simulink model "bldc_new_good"  (R2018a)
settings: Solver=FixedStepDiscrete  StartTime=0.0  StopTime=t_l+0.5  RelTol=1e-3  EnableMultiTasking=on
PreLoadFcn:
  | Ts=2e-6;
values from neighbouring files (symbols this model uses):
  r1 = -0.136    [Platforma_algorytm.m]
  r2 = -0.04    [Platforma_algorytm.m]
  t_l = length(right_foot)*dt    [Platforma_algorytm.m]
  t_r = length(left_foot)*dt    [Platforma_algorytm.m]
  w_x = ((60*v*4.29)/r1)/(2*pi*10)    [Platforma_algorytm.m]
  w_y = ((60*v*4.29)/r2)/(2*pi*10)    [Platforma_algorytm.m]
undefined symbols (not defined in the file or in its folder): DiscIntNeverNeededParam, s
libraries: powerlib_meascontrol x4, powerlib x3, electricdrivelib x2, AC7DriveInternalModels x2, simulink x1
Description:
  | Copyright 2008-2018 The MathWorks, Inc.
settings Model: ExtModeAutoUpdateStatusClock=off  Creator=MathWorks  LastModifiedBy=cinek
settings SolverCC: AutoInsertRateTranBlk=on
settings DataIOCC: LimitDataPoints=on  SaveFormat=Array  SignalLoggingSaveFormat=ModelDataLogs  SignalLoggingName=sigsOut
settings OptimizationCC: ExpressionDepthLimit=2147483647  InitFltsAndDblsToZero=on  LifeSpan=inf
settings DebuggingCC: UnderspecifiedInitializationDetection=Classic  MergeDetectMultiDrivingBlocksExec=none  CheckExecutionContextPreStartOutputMsg=on  CheckExecutionContextRuntimeOutputMsg=on  SignalResolutionControl=TryResolveAllWithWarning  MultiTaskDSMMsg=warning  MultiTaskCondExecSysMsg=none  FcnCallInpInsideContextMsg=warning  UnconnectedLineMsg=none  StateNameClashWarn=warning  SFUnexpectedBacktrackingDiag=warning  SFNoUnconditionalDefaultTransitionDiag=warning  SFExecutionAtInitializationDiag=none
settings HardwareCC: ProdBitPerPointer=32  ProdBitPerSizeT=32  ProdBitPerPtrDiffT=32  ProdLargestAtomicFloat=None  ProdIntDivRoundTo=Undefined  ProdEndianess=Unspecified  ProdWordSize=32  ProdHWDeviceType=32-bit Generic  TargetUnknown=on
settings ModelReferenceCC: PropagateSignalLabelsOutOfModel=off
settings CodeAppCC: StateflowObjectComments=on
settings GRTTargetCC: TargetLangStandard=C89/C90 (ANSI)  GeneratePreprocessorConditionals=Disable all  CombineOutputUpdateFcns=off  GRTInterface=on
settings ConfigComp: CovMetricSettings=dw  CovHtmlReporting=on  CovSaveCumulativeToWorkspaceVar=on  CovSaveSingleToWorkspaceVar=on  CovExternalEMLEnable=off  CovSFcnEnable=off
settings SimscapeCC: SimscapeNormalizeSystem=off

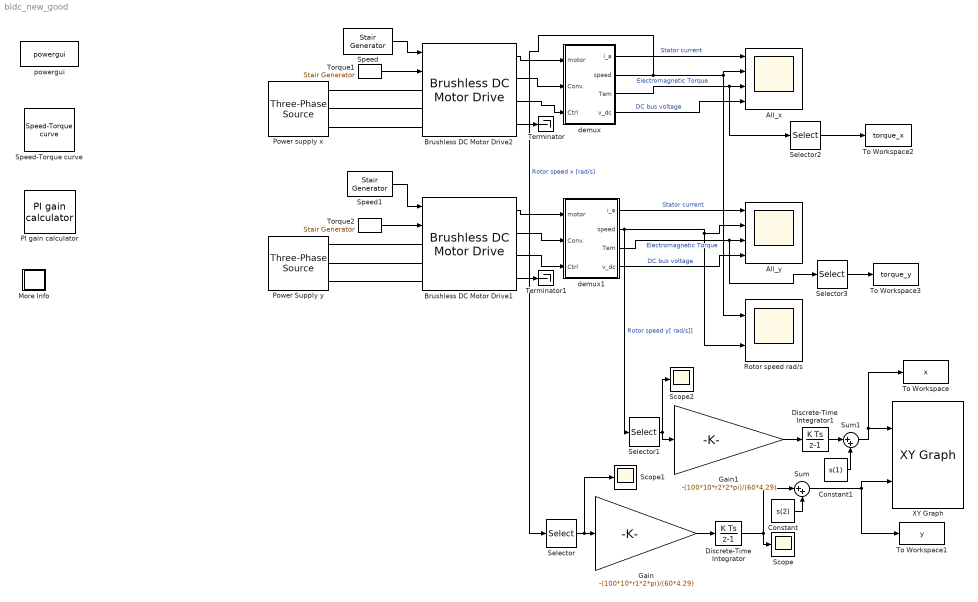
== system bldc_new_good ==
  All_x : Scope  NumInputPorts=4
  All_y : Scope  NumInputPorts=4
  Brushless DC Motor Drive1 : electricdrivelib/AC drives/Brushless DC Motor Drive  Rs=0.2  Lls=8.5e-3  Flat=120  MachineConstant=Flux linkage established by magnets (V.s)  FluxCst=0.175  VoltageCst=146.6077  TorqueCst=1.4  ia=0  ib=0  J=0.089  Friction=0.005  p=4  wm=0  thetam=0  Rsnb_rec=10e3  Csnb_rec=20e-9  Ron_rec=1e-3  Vf_rec=1.3  cap_bus=2000e-6  Rbrake=8  fbrake=4000  activationVoltage=0  shutdownVoltage=50  deviceType=IGBT / Diodes  Ron_inv=1e-3  Vf_inv=0.8  Vfd_inv=0.8  Tf=1e-6  Tt=2e-6  Tf_GTO=10e-6  Tt_GTO=20e-6  Rsnb_inv=5000  Csnb_inv=inf  regulationType=Speed regulation  Acc=1000  Dec=-1000  kp_sc=3.3  ki_sc=300  fc_sc=285  Tsc=140e-6  Tmin=-17.8  Tmax=17.8  h=0.01  freq_max=20e3  Tvect=20e-6  baseSampleTime=2e-06  outputBusMode=Multiple output buses  busLabels=off  MechanicalLoad=Torque Tm  modelDetailLevel=Detailed  driveType=AC7  AverageValue=off
      settings: SourceProductName=Simscape Power Systems  SourceProductBaseCode=PS
  Brushless DC Motor Drive2 : electricdrivelib/AC drives/Brushless DC Motor Drive  Rs=0.2  Lls=8.5e-3  Flat=120  MachineConstant=Flux linkage established by magnets (V.s)  FluxCst=0.175  VoltageCst=146.6077  TorqueCst=1.4  ia=0  ib=0  J=0.089  Friction=0.005  p=4  wm=0  thetam=0  Rsnb_rec=10e3  Csnb_rec=20e-9  Ron_rec=1e-3  Vf_rec=1.3  cap_bus=2000e-6  Rbrake=8  fbrake=4000  activationVoltage=0  shutdownVoltage=80  deviceType=IGBT / Diodes  Ron_inv=1e-3  Vf_inv=0.8  Vfd_inv=0.8  Tf=1e-6  Tt=2e-6  Tf_GTO=10e-6  Tt_GTO=20e-6  Rsnb_inv=5000  Csnb_inv=inf  regulationType=Speed regulation  Acc=1000  Dec=-1000  kp_sc=3.3  ki_sc=300  fc_sc=285  Tsc=140e-6  Tmin=-17.8  Tmax=17.8  h=0.01  freq_max=20e3  Tvect=20e-6  baseSampleTime=2e-06  outputBusMode=Multiple output buses  busLabels=off  MechanicalLoad=Torque Tm  modelDetailLevel=Average  driveType=AC7  AverageValue=on
      settings: SourceProductName=Simscape Power Systems  SourceProductBaseCode=PS
  Constant : Constant  Value=s(2)
  Constant1 : Constant  Value=s(1)
  Discrete-Time Integrator : DiscreteIntegrator  SampleTime=1/60  ICPrevOutput=DiscIntNeverNeededParam  ICPrevScaledInput=DiscIntNeverNeededParam
  Discrete-Time Integrator1 : DiscreteIntegrator  SampleTime=1/60  ICPrevOutput=DiscIntNeverNeededParam  ICPrevScaledInput=DiscIntNeverNeededParam
  Gain : Gain  Gain=-(100*10*r1*2*pi)/(60*4.29)
  Gain1 : Gain  Gain=-(100*10*r2*2*pi)/(60*4.29)
  More Info : Subsystem
      settings: OpenFcn=showdemo(bdroot(gcb))
      mask Display: disp('?')
  PI gain calculator : AC7DriveInternalModels/PI gain calculator  mec=[0.089 0.005 4]  specs=on  ele=[0.2 8.5e-3]  lam=0.175  open_loop=off  zeta=0.99  Trd=0.13/5  check=off
  Power Supply y : powerlib/Electrical Sources/Three-Phase Source  InternalConnection=Yn  VoltagePhases=off  Voltage=20  PhaseAngle=0  Voltage_phases=[25e3 25e3 25e3]/sqrt(3)  PhaseAngles_phases=[0 -120 +120]  Frequency=60  NonIdealSource=on  SpecifyImpedance=off  Resistance=0.02  Inductance=0.05e-3  ShortCircuitLevel=100e6  BaseVoltage=25e3  XRratio=7  BusType=swing  Pref=0  Qref=0  Prefabc=[10e3, 10e3, 10e3]  Qrefabc=[0, 0, 0]  Qmin=-inf  Qmax=inf
  Power supply x : powerlib/Electrical Sources/Three-Phase Source  InternalConnection=Yn  VoltagePhases=off  Voltage=30  PhaseAngle=0  Voltage_phases=[25e3 25e3 25e3]/sqrt(3)  PhaseAngles_phases=[0 -120 +120]  Frequency=60  NonIdealSource=on  SpecifyImpedance=off  Resistance=0.02  Inductance=0.05e-3  ShortCircuitLevel=100e6  BaseVoltage=25e3  XRratio=7  BusType=swing  Pref=0  Qref=0  Prefabc=[10e3, 10e3, 10e3]  Qrefabc=[0, 0, 0]  Qmin=-inf  Qmax=inf
  Rotor speed rad/s : Scope  NumInputPorts=2
  Scope : Scope
  Scope1 : Scope
  Scope2 : Scope
  Selector : Selector  NumberOfDimensions=2  InputPortWidth=3  IndexOptions=Index vector (dialog),Index vector (dialog)  Indices=[1],1  OutputSizes=1,1
  Selector1 : Selector  NumberOfDimensions=2  InputPortWidth=3  IndexOptions=Index vector (dialog),Index vector (dialog)  Indices=[1],1  OutputSizes=1,1
  Selector2 : Selector  NumberOfDimensions=2  InputPortWidth=3  IndexOptions=Index vector (dialog),Index vector (dialog)  Indices=[2],1  OutputSizes=1,1
  Selector3 : Selector  NumberOfDimensions=2  InputPortWidth=2  IndexOptions=Index vector (dialog),Select all  Indices=2,1  OutputSizes=1,1
  Speed : powerlib_meascontrol/Pulse & Signal Generators/Stair Generator  t=[0 t_r]  e=[w_x 0]  Ts=Ts
      settings: SourceProductName=Simscape Power Systems
  Speed-Torque curve : AC7DriveInternalModels/Speed-Torque curve  ele=[0.2 8.5e-3]  Flux=0.175  mec=[0.089 0.005 4]  Vdc=310  Tmax=17.8  accel=1000  check=off
  Speed1 : powerlib_meascontrol/Pulse & Signal Generators/Stair Generator  t=[0 t_l]  e=[w_y 0]  Ts=Ts
      settings: SourceProductName=Simscape Power Systems
  Sum : Sum  Inputs=|++
  Sum1 : Sum  Inputs=|++
  Terminator : Terminator
  Terminator1 : Terminator
  To Workspace : ToWorkspace  VariableName=x  SampleTime=-1
      settings: Save2DSignal=2-D array (concatenate along first dimension)
  To Workspace1 : ToWorkspace  VariableName=y  SampleTime=-1
      settings: Save2DSignal=2-D array (concatenate along first dimension)
  To Workspace2 : ToWorkspace  VariableName=torque_x  SaveFormat=Structure With Time  SampleTime=-1
      settings: Save2DSignal=2-D array (concatenate along first dimension)
  To Workspace3 : ToWorkspace  VariableName=torque_y  SaveFormat=Structure With Time  SampleTime=-1
      settings: Save2DSignal=2-D array (concatenate along first dimension)
  Torque1 : powerlib_meascontrol/Pulse & Signal Generators/Stair Generator  t=[0 t_r]  e=[8 -8]  Ts=Ts
      settings: SourceProductName=Simscape Power Systems
  Torque2 : powerlib_meascontrol/Pulse & Signal Generators/Stair Generator  t=[0 t_r]  e=[3 -3]  Ts=Ts
      settings: SourceProductName=Simscape Power Systems
  XY Graph : simulink/Sinks/XY Graph  xmin=-100  xmax=100  ymin=-100  ymax=100  st=1/60
  demux : Subsystem
  demux1 : Subsystem
  powergui : powerlib/powergui  SimulationMode=Discrete  SampleTime=Ts  frequency=60  Iterations=50  frequencyindice=0  Pbase=100e6  ErrMax=1e-4  UnitsV=kV  UnitsW=MW  buscounter=0  FunctionMessages=off  echomessages=off  EnableUseOfTLC=off  CurrentSourceSwitches=off  DisableSnubberDevices=off  DisableRonSwitches=off  DisableVfSwitches=off  DisplayEquations=off  SolverType=Tustin/Backward Euler (TBE)  Interpol=off  ExternalGateDelay=off  methode=off  Ts=0  x0status=blocks  SPID=off  SwTol=0  HookPort=off  RestoreLinks=warning  ResistiveCurrentMeasurement=off  Frange=[0:2:500]  Ylog=off  Xlog=on  ShowGrid=off  save=off  variable=ZData  structure=0  ZoomFFT=on  StartTime=0.0  cycles=1  DisplayStyle=1  fundamental=60  FreqAxis=off  MaxFrequency=1000  frequencyindicesteady=1  RmsSteady=1  display=off
  wires:
  Brushless DC Motor Drive2/1 -> demux/1(motor)
  demux/1(i_a) -> All_x/1  "Stator current"
  demux/2(speed) -> Selector/1, All_x/2, Rotor speed rad/s/1  "Rotor speed x [rad/s]"
  demux/3(Tem) -> Selector2/1, All_x/3  "Electromagnetic Torque"
  demux/4(v_dc) -> All_x/4  "DC bus voltage"
  demux1/3(Tem) -> Selector3/1, All_y/3  "Electromagnetic Torque"
  Brushless DC Motor Drive1/3 -> demux1/3(Ctrl)
  demux1/4(v_dc) -> All_y/4  "DC bus voltage"
  Brushless DC Motor Drive1/1 -> demux1/1(motor)
  demux1/1(i_a) -> All_y/1  "Stator current"
  Brushless DC Motor Drive1/2 -> demux1/2(Conv.)
  demux1/2(speed) -> Rotor speed rad/s/2, All_y/2, Selector1/1  "Rotor speed y[ rad/s]]"
  Brushless DC Motor Drive2/2 -> demux/2(Conv.)
  Brushless DC Motor Drive2/3 -> demux/3(Ctrl)
  Selector1/1 -> Gain1/1, Scope2/1
  Discrete-Time Integrator/1 -> Sum/1, Scope/1
  Discrete-Time Integrator1/1 -> Sum1/1
  Gain1/1 -> Discrete-Time Integrator1/1
  Sum/1 -> XY Graph/2, To Workspace1/1
  Constant/1 -> Sum/2
  Sum1/1 -> To Workspace/1, XY Graph/1
  Constant1/1 -> Sum1/2
  Gain/1 -> Discrete-Time Integrator/1
  Selector3/1 -> To Workspace3/1
  Selector2/1 -> To Workspace2/1
  Speed1/1 -> Brushless DC Motor Drive1/1
  Speed/1 -> Brushless DC Motor Drive2/1
  Brushless DC Motor Drive2/4 -> Terminator/1
  Brushless DC Motor Drive1/4 -> Terminator1/1
  Torque1/1 -> Brushless DC Motor Drive2/2
  Torque2/1 -> Brushless DC Motor Drive1/2
  Selector/1 -> Scope1/1, Gain/1
  connections:
  Brushless DC Motor Drive2/LConn1 -- Power supply x/RConn1
  Brushless DC Motor Drive2/LConn2 -- Power supply x/RConn2
  Brushless DC Motor Drive2/LConn3 -- Power supply x/RConn3
  Power Supply y/RConn1 -- Brushless DC Motor Drive1/LConn1
  Power Supply y/RConn2 -- Brushless DC Motor Drive1/LConn2
  Power Supply y/RConn3 -- Brushless DC Motor Drive1/LConn3

== system bldc_new_good/More Info ==

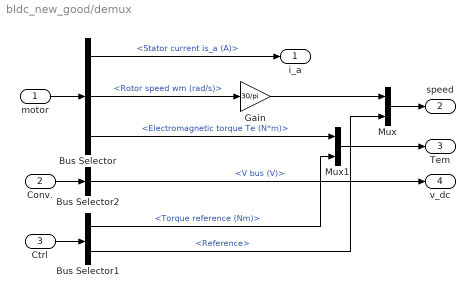
== system bldc_new_good/demux ==
  motor : Inport
  Conv. : Inport  Port=2
  Ctrl : Inport  Port=3
  Bus Selector : BusSelector  OutputSignals=Stator current is_a (A),Rotor speed wm (rad/s),Electromagnetic torque Te (N*m)
  Bus Selector1 : BusSelector  OutputSignals=Torque reference (Nm),Reference
  Bus Selector2 : BusSelector  OutputSignals=V bus (V)
  Gain : Gain  Gain=30/pi  SaturateOnIntegerOverflow=on  OutDataTypeStr=Inherit: Same as input  ParamDataTypeStr=Inherit: Same as input
  Mux : Mux  Inputs=2
  Mux1 : Mux  Inputs=2
  i_a : Outport
  speed : Outport  Port=2
  Tem : Outport  Port=3
  v_dc : Outport  Port=4
  wires:
  Bus Selector/2 -> Gain/1  "<Rotor speed wm (rad/s)>"
  Bus Selector2/1 -> v_dc/1  "<V bus (V)>"
  Conv./1 -> Bus Selector2/1
  Ctrl/1 -> Bus Selector1/1
  Bus Selector1/1 -> Mux1/2  "<Torque reference (Nm)>"
  Bus Selector1/2 -> Mux/2  "<Reference>"
  Gain/1 -> Mux/1
  Bus Selector/1 -> i_a/1  "<Stator current is_a (A)>"
  Bus Selector/3 -> Mux1/1  "<Electromagnetic torque Te (N*m)>"
  Mux1/1 -> Tem/1
  Mux/1 -> speed/1
  motor/1 -> Bus Selector/1

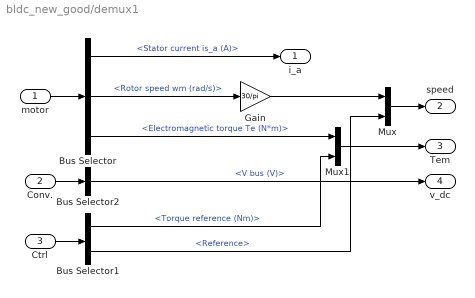
== system bldc_new_good/demux1 ==
  motor : Inport
  Conv. : Inport  Port=2
  Ctrl : Inport  Port=3
  Bus Selector : BusSelector  OutputSignals=Stator current is_a (A),Rotor speed wm (rad/s),Electromagnetic torque Te (N*m)
  Bus Selector1 : BusSelector  OutputSignals=Torque reference (Nm),Reference
  Bus Selector2 : BusSelector  OutputSignals=V bus (V)
  Gain : Gain  Gain=30/pi  SaturateOnIntegerOverflow=on  OutDataTypeStr=Inherit: Same as input  ParamDataTypeStr=Inherit: Same as input
  Mux : Mux  Inputs=2
  Mux1 : Mux  Inputs=2
  i_a : Outport
  speed : Outport  Port=2
  Tem : Outport  Port=3
  v_dc : Outport  Port=4
  wires:
  Bus Selector/2 -> Gain/1  "<Rotor speed wm (rad/s)>"
  Bus Selector2/1 -> v_dc/1  "<V bus (V)>"
  Conv./1 -> Bus Selector2/1
  Ctrl/1 -> Bus Selector1/1
  Bus Selector1/1 -> Mux1/2  "<Torque reference (Nm)>"
  Bus Selector1/2 -> Mux/2  "<Reference>"
  Gain/1 -> Mux/1
  Bus Selector/1 -> i_a/1  "<Stator current is_a (A)>"
  Bus Selector/3 -> Mux1/1  "<Electromagnetic torque Te (N*m)>"
  Mux1/1 -> Tem/1
  Mux/1 -> speed/1
  motor/1 -> Bus Selector/1
